simulink model "test_stimulation_visual_movie"  (Simulink 4.00)
settings: Solver=FixedStepDiscrete  SolverMode=SingleTasking  StartTime=0.0  StopTime=24  FixedStep=0.05  RelTol=1e-3
libraries: simulink3 x1, stimulation_visual_lib x1
settings Model: LastModifiedBy=bsaunder

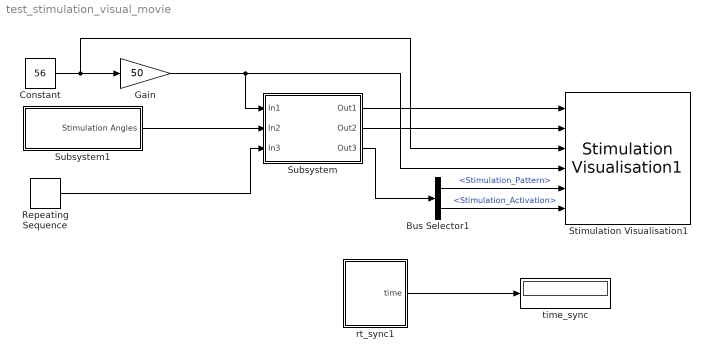
== system test_stimulation_visual_movie ==
  Bus Selector1 : BusSelector  OutputSignals=Stimulation_Pattern,Stimulation_Activation  MuxedOutput=off
  Constant : Constant  Value=56
  Gain : Gain  Gain=50  Multiplication=Element-wise(K.*u)  SaturateOnIntegerOverflow=on
  Repeating Sequence : simulink3/Sources/Repeating Sequence  rep_seq_t=[0 1 1.5 2 3]  rep_seq_y=[0.0 0.25 0.5 1.0 1.0]
  Stimulation Visualisation1 : stimulation_visual_lib/Stimulation Visualisation1  show=on  Ts=0.05
  Subsystem : Subsystem
      settings: RTWFcnNameOpts=Auto  RTWFileNameOpts=Auto
  Subsystem1 : Subsystem
      settings: RTWFcnNameOpts=Auto  RTWFileNameOpts=Auto
  rt_sync1 : Subsystem  mask{Ts=0.05}
      mask prompts: Ts "Sample Time"
      settings: RTWFcnNameOpts=Auto  RTWFileNameOpts=Auto
      mask Display: fprintf('Real\n Time\n sync')
  time_sync : Display
      settings: Format=short
  wires:
  Repeating Sequence/1 -> Subsystem/3(In3)
  Subsystem1/1(Stimulation Angles) -> Subsystem/2(In2)
  Constant/1 -> Gain/1, Stimulation Visualisation1/3
  Gain/1 -> Subsystem/1(In1), Stimulation Visualisation1/4
  Bus Selector1/1 -> Stimulation Visualisation1/5  "<Stimulation_Pattern>"
  Bus Selector1/2 -> Stimulation Visualisation1/6  "<Stimulation_Activation>"
  Subsystem/3(Out3) -> Bus Selector1/1
  Subsystem/1(Out1) -> Stimulation Visualisation1/1
  Subsystem/2(Out2) -> Stimulation Visualisation1/2
  rt_sync1/1(time) -> time_sync/1

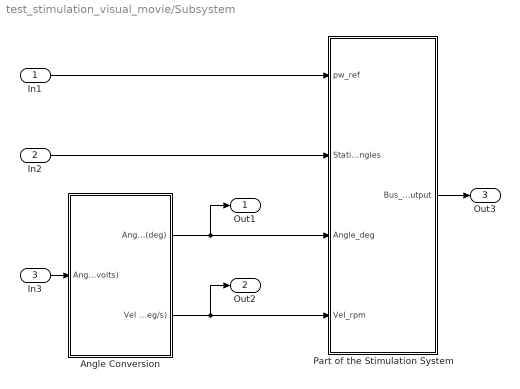
== system test_stimulation_visual_movie/Subsystem ==
  In1 : Inport  Port=1  LatchInput=off
  In2 : Inport  Port=2  LatchInput=off
  In3 : Inport  Port=3  LatchInput=off
  Angle Conversion : Subsystem
      settings: RTWFcnNameOpts=Auto  RTWFileNameOpts=Auto
  Part of the Stimulation System : Subsystem
      settings: RTWFcnNameOpts=Auto  RTWFileNameOpts=Auto
  Out1 : Outport  Port=1
  Out2 : Outport  Port=2
  Out3 : Outport  Port=3
  wires:
  Angle Conversion/1(Angle (deg)) -> Part of the Stimulation System/3(Angle_deg), Out1/1
  Angle Conversion/2(Vel (deg/s)) -> Part of the Stimulation System/4(Vel_rpm), Out2/1
  Part of the Stimulation System/1(Bus_Output) -> Out3/1
  In1/1 -> Part of the Stimulation System/1(pw_ref)
  In2/1 -> Part of the Stimulation System/2(Static Stimulation Angles)
  In3/1 -> Angle Conversion/1(Angle (0 to 1 volts))

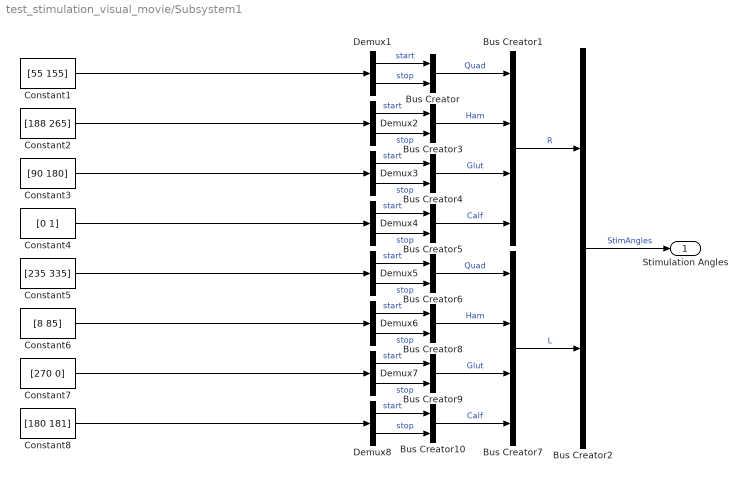
== system test_stimulation_visual_movie/Subsystem1 ==
  Bus Creator{,2..6,8..10} (9 alike) : BusCreator  Inputs=2
  Bus Creator1 : BusCreator  Inputs=4
  Bus Creator7 : BusCreator  Inputs=4
  Constant1 : Constant  Value=[55 155]
  Constant2 : Constant  Value=[188 265]
  Constant3 : Constant  Value=[90 180]
  Constant4 : Constant  Value=[0 1]
  Constant5 : Constant  Value=[235 335]
  Constant6 : Constant  Value=[8 85]
  Constant7 : Constant  Value=[270 0]
  Constant8 : Constant  Value=[180 181]
  Demux{1..8} (8 alike) : Demux  Outputs=2  BusSelectionMode=off
  Stimulation Angles : Outport  Port=1
  wires:
  Bus Creator7/1 -> Bus Creator2/2  "L"
  Constant8/1 -> Demux8/1
  Constant7/1 -> Demux7/1
  Constant6/1 -> Demux6/1
  Constant5/1 -> Demux5/1
  Bus Creator10/1 -> Bus Creator7/4  "Calf"
  Bus Creator9/1 -> Bus Creator7/3  "Glut"
  Bus Creator8/1 -> Bus Creator7/2  "Ham"
  Demux8/2 -> Bus Creator10/2  "stop"
  Demux8/1 -> Bus Creator10/1  "start"
  Demux7/2 -> Bus Creator9/2  "stop"
  Demux7/1 -> Bus Creator9/1  "start"
  Demux6/2 -> Bus Creator8/2  "stop"
  Demux6/1 -> Bus Creator8/1  "start"
  Bus Creator6/1 -> Bus Creator7/1  "Quad"
  Demux5/2 -> Bus Creator6/2  "stop"
  Demux5/1 -> Bus Creator6/1  "start"
  Constant4/1 -> Demux4/1
  Constant3/1 -> Demux3/1
  Constant2/1 -> Demux2/1
  Bus Creator5/1 -> Bus Creator1/4  "Calf"
  Bus Creator4/1 -> Bus Creator1/3  "Glut"
  Bus Creator3/1 -> Bus Creator1/2  "Ham"
  Demux4/2 -> Bus Creator5/2  "stop"
  Demux4/1 -> Bus Creator5/1  "start"
  Demux3/2 -> Bus Creator4/2  "stop"
  Demux3/1 -> Bus Creator4/1  "start"
  Demux2/2 -> Bus Creator3/2  "stop"
  Demux2/1 -> Bus Creator3/1  "start"
  Bus Creator1/1 -> Bus Creator2/1  "R"
  Bus Creator/1 -> Bus Creator1/1  "Quad"
  Demux1/2 -> Bus Creator/2  "stop"
  Demux1/1 -> Bus Creator/1  "start"
  Constant1/1 -> Demux1/1
  Bus Creator2/1 -> Stimulation Angles/1  "StimAngles"

== system test_stimulation_visual_movie/rt_sync1 ==
  S-Function : S-Function  FunctionName=sf_rtsync  Parameters=Ts  PortCounts=[]  SFunctionModules=''
  time : Outport  Port=1
  wires:
  S-Function/1 -> time/1

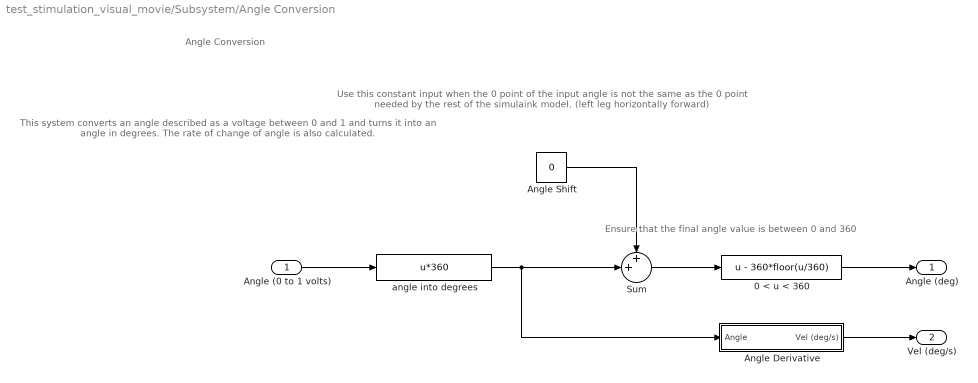
== system test_stimulation_visual_movie/Subsystem/Angle Conversion ==
  note: Angle Conversion
  note: Use this constant input
      | when the 0 point of the
      | input angle is not the same
      | as the 0 point needed by
      | the rest of the simulaink
      | model.
      | (left leg horizontally forward)
  note: Ensure that the final angle
      | value is between 0 and 360
  note: This system converts an
      | angle described as a voltage
      | between 0 and 1 and turns it
      | into an angle in degrees.
      | The rate of change of angle
      | is also calculated.
  Angle (0 to 1 volts) : Inport  Port=1  LatchInput=off
  0 < u < 360 : Fcn  Expr=u - 360*floor(u/360)
  Angle Derivative : Subsystem  mask(AngleDer){Tdf=0.5, Ts=0.05}
      mask prompts: Tdf "Filter constant"; Ts "Sampling Time"
      mask help:
      | This block calculates the angular velocity from the angle measuremet.  If the input angle is in degrees then the output velocity is in deg/s.  The block takes account of the transition from 359 deg to 0 deg or vice versa and computes the derivative based on the sample time given  The output is passed through a low pass filter based on the fliter constant also given.
      |
      | Implemented by Nils-Otto Negaard
      | Documented by Ben Saunders (17/06/2003)
      settings: RTWFcnNameOpts=Auto  RTWFileNameOpts=Auto
  Angle Shift : Constant  Value=0
  Sum : Sum  Inputs=++|  SaturateOnIntegerOverflow=on
  angle into degrees : Fcn  Expr=u*360
  Angle (deg) : Outport  Port=1
  Vel (deg/s) : Outport  Port=2
  wires:
  Angle Shift/1 -> Sum/1
  Angle Derivative/1(Vel (deg/s)) -> Vel (deg/s)/1
  Angle (0 to 1 volts)/1 -> angle into degrees/1
  0 < u < 360/1 -> Angle (deg)/1
  Sum/1 -> 0 < u < 360/1
  angle into degrees/1 -> Sum/2, Angle Derivative/1(Angle)

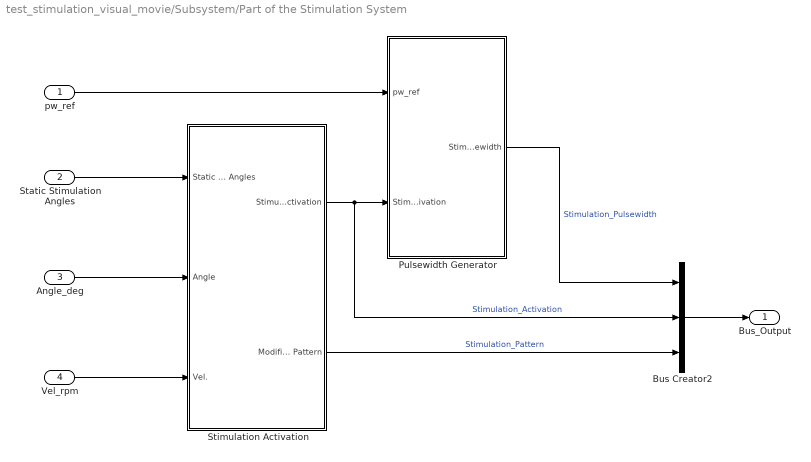
== system test_stimulation_visual_movie/Subsystem/Part of the Stimulation System ==
  pw_ref : Inport  Port=1  LatchInput=off
  Static Stimulation Angles : Inport  Port=2  LatchInput=off
  Angle_deg : Inport  Port=3  LatchInput=off
  Vel_rpm : Inport  Port=4  LatchInput=off
  Bus Creator2 : BusCreator  Inputs=3
  Pulsewidth Generator : Subsystem
      settings: RTWFcnNameOpts=Auto  RTWFileNameOpts=Auto
  Stimulation Activation : Subsystem
      settings: RTWFcnNameOpts=Auto  RTWFileNameOpts=Auto
  Bus_Output : Outport  Port=1
  wires:
  Bus Creator2/1 -> Bus_Output/1
  pw_ref/1 -> Pulsewidth Generator/1(pw_ref)
  Stimulation Activation/2(Modified Stimulation Pattern) -> Bus Creator2/3  "Stimulation_Pattern"
  Pulsewidth Generator/1(Stimulation Pulsewidth) -> Bus Creator2/1  "Stimulation_Pulsewidth"
  Vel_rpm/1 -> Stimulation Activation/3(Vel.)
  Angle_deg/1 -> Stimulation Activation/2(Angle)
  Static Stimulation Angles/1 -> Stimulation Activation/1(Static Stimulation Angles)
  Stimulation Activation/1(Stimulation Activation) -> Bus Creator2/2, Pulsewidth Generator/2(Stimulation Activation)  "Stimulation_Activation"

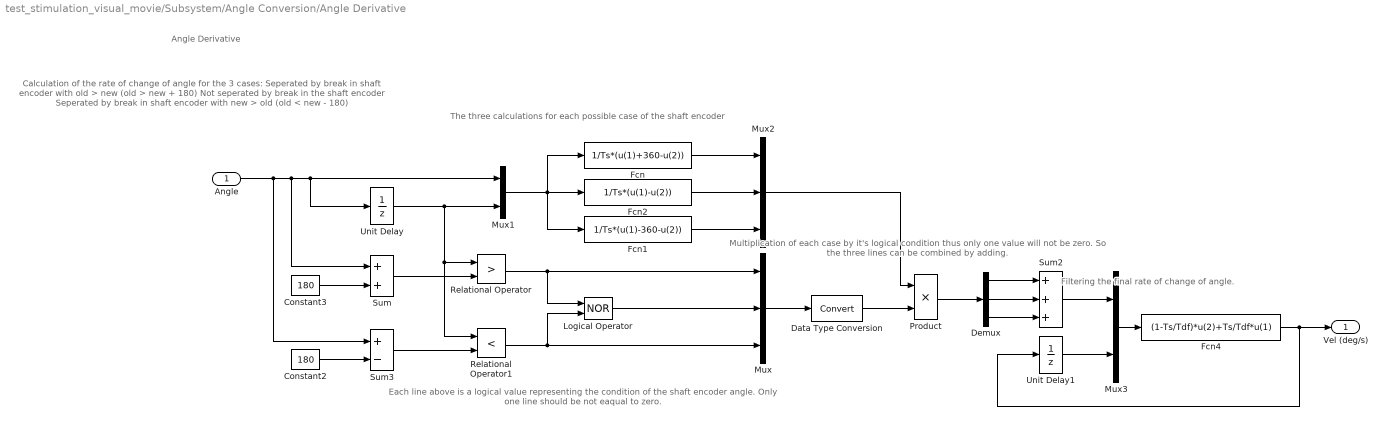
== system test_stimulation_visual_movie/Subsystem/Angle Conversion/Angle Derivative ==
  note: Angle Derivative
  note: Filtering the final rate of
      | change of angle.
  note: Multiplication of each case
      | by it's logical condition thus
      | only one value will not be zero.
      | So the three lines can be
      | combined by adding.
  note: The three calculations for each
      | possible case of the shaft encoder
  note: Each line above is a logical value
      | representing the condition of the
      | shaft encoder angle.  Only one line
      | should be not eaqual to zero.
  note: Calculation of the rate of change of angle
      | for the 3 cases:
      | Seperated by break in shaft encoder with old > new (old > new + 180)
      | Not seperated by break in the shaft encoder
      | Seperated by break in shaft encoder with new > old (old < new - 180)
  Angle : Inport  Port=1  LatchInput=off
  Constant2 : Constant  Value=180  VectorParams1D=off
  Constant3 : Constant  Value=180  VectorParams1D=off
  Data Type Conversion : DataTypeConversion  DataType=double  SaturateOnIntegerOverflow=on
  Demux : Demux  Outputs=3  BusSelectionMode=off
  Fcn : Fcn  Expr=1/Ts*(u(1)+360-u(2))
  Fcn1 : Fcn  Expr=1/Ts*(u(1)-360-u(2))
  Fcn2 : Fcn  Expr=1/Ts*(u(1)-u(2))
  Fcn4 : Fcn  Expr=(1-Ts/Tdf)*u(2)+Ts/Tdf*u(1)
  Logical Operator : Logic  Operator=NOR  Inputs=2
  Mux : Mux  Inputs=3
  Mux1 : Mux  Inputs=2
  Mux2 : Mux  Inputs=3
  Mux3 : Mux  Inputs=2
  Product : Product  Inputs=2  Multiplication=Element-wise(.*)  SaturateOnIntegerOverflow=on
  Relational Operator : RelationalOperator  Operator=>
  Relational Operator1 : RelationalOperator  Operator=<
  Sum : Sum  Inputs=++  SaturateOnIntegerOverflow=on
  Sum2 : Sum  Inputs=+++  SaturateOnIntegerOverflow=on
  Sum3 : Sum  Inputs=+-  SaturateOnIntegerOverflow=on
  Unit Delay : UnitDelay  X0=0  SampleTime=0.05
      settings: RTWStateStorageClass=Auto
  Unit Delay1 : UnitDelay  X0=0  SampleTime=Ts
      settings: RTWStateStorageClass=Auto
  Vel (deg/s) : Outport  Port=1
  wires:
  Fcn1/1 -> Mux2/3
  Fcn2/1 -> Mux2/2
  Logical Operator/1 -> Mux/2
  Sum3/1 -> Relational Operator1/2
  Constant3/1 -> Sum/2
  Angle/1 -> Unit Delay/1, Mux1/1, Sum/1, Sum3/1
  Sum2/1 -> Mux3/1
  Demux/3 -> Sum2/3
  Demux/2 -> Sum2/2
  Demux/1 -> Sum2/1
  Product/1 -> Demux/1
  Unit Delay1/1 -> Mux3/2
  Mux3/1 -> Fcn4/1
  Fcn4/1 -> Vel (deg/s)/1, Unit Delay1/1
  Mux2/1 -> Product/1
  Fcn/1 -> Mux2/1
  Mux1/1 -> Fcn2/1, Fcn1/1, Fcn/1
  Mux/1 -> Data Type Conversion/1
  Relational Operator/1 -> Mux/1, Logical Operator/1
  Relational Operator1/1 -> Mux/3, Logical Operator/2
  Constant2/1 -> Sum3/2
  Sum/1 -> Relational Operator/2
  Unit Delay/1 -> Relational Operator/1, Relational Operator1/1, Mux1/2
  Data Type Conversion/1 -> Product/2

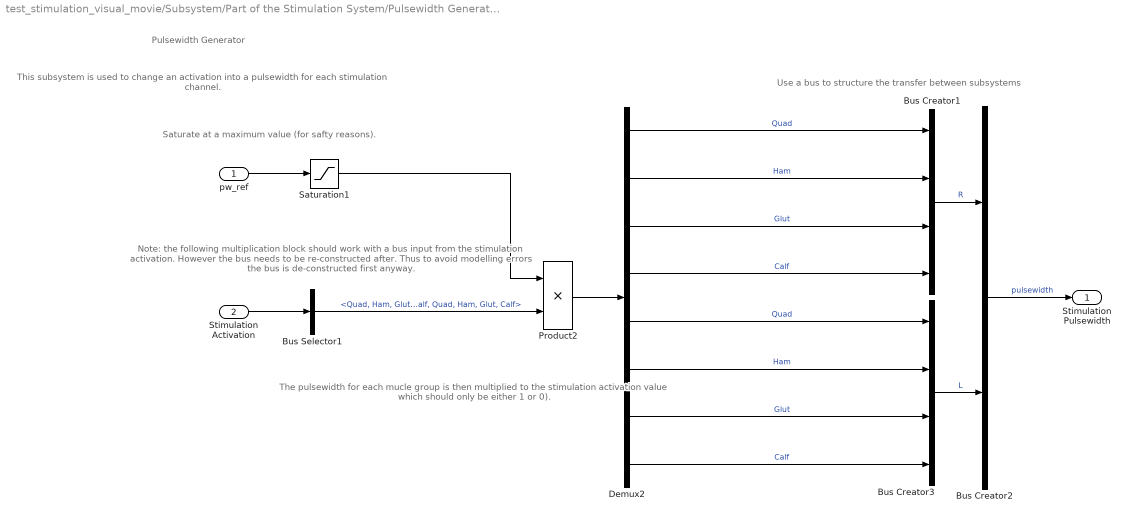
== system test_stimulation_visual_movie/Subsystem/Part of the Stimulation System/Pulsewidth Generator ==
  note: The pulsewidth for each
      | mucle group is then
      | multiplied to the stimulation
      | activation value which
      | should only be either 1 or 0).
  note: Use a bus to structure the
      | transfer between subsystems
  note: Note: the following multiplication
      | block should work with a bus input
      | from the stimulation activation.
      | However the bus needs to be
      | re-constructed after.  Thus to
      | avoid modelling errors the bus is
      | de-constructed first anyway.
  note: This subsystem is used to change
      | an activation into a pulsewidth for
      | each stimulation channel.
  note: Pulsewidth Generator
  note: Saturate at a maximum
      | value (for safty reasons).
  pw_ref : Inport  Port=1  LatchInput=off
  Stimulation Activation : Inport  Port=2  LatchInput=off
  Bus Creator1 : BusCreator  Inputs=4
  Bus Creator2 : BusCreator  Inputs=2
  Bus Creator3 : BusCreator  Inputs=4
  Bus Selector1 : BusSelector  OutputSignals=R.Quad,R.Ham,R.Glut,R.Calf,L.Quad,L.Ham,L.Glut,L.Calf  MuxedOutput=on
  Demux2 : Demux  Outputs=8  BusSelectionMode=off
  Product2 : Product  Inputs=2  Multiplication=Element-wise(.*)  SaturateOnIntegerOverflow=on
  Saturation1 : Saturate  UpperLimit=510  LowerLimit=0  LinearizeAsGain=on
  Stimulation Pulsewidth : Outport  Port=1
  wires:
  Saturation1/1 -> Product2/1
  pw_ref/1 -> Saturation1/1
  Product2/1 -> Demux2/1
  Bus Selector1/1 -> Product2/2  "<Quad, Ham, Glut, Calf, Quad, Ham, Glut, Calf>"
  Bus Creator2/1 -> Stimulation Pulsewidth/1  "pulsewidth"
  Bus Creator3/1 -> Bus Creator2/2  "L"
  Bus Creator1/1 -> Bus Creator2/1  "R"
  Demux2/1 -> Bus Creator1/1  "Quad"
  Demux2/2 -> Bus Creator1/2  "Ham"
  Demux2/3 -> Bus Creator1/3  "Glut"
  Demux2/4 -> Bus Creator1/4  "Calf"
  Demux2/5 -> Bus Creator3/1  "Quad"
  Demux2/6 -> Bus Creator3/2  "Ham"
  Demux2/7 -> Bus Creator3/3  "Glut"
  Demux2/8 -> Bus Creator3/4  "Calf"
  Stimulation Activation/1 -> Bus Selector1/1

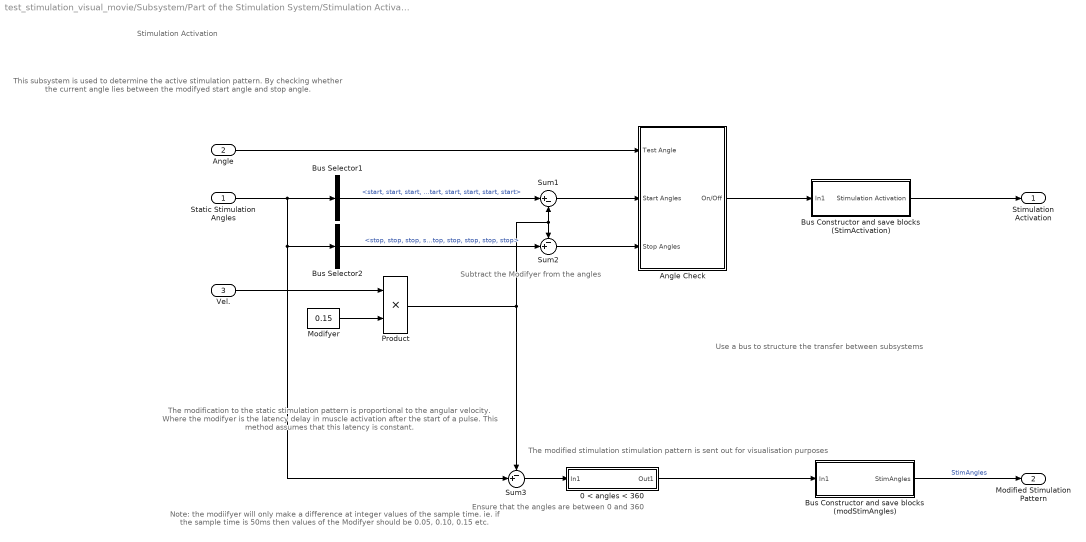
== system test_stimulation_visual_movie/Subsystem/Part of the Stimulation System/Stimulation Activation ==
  note: Use a bus to structure the
      | transfer between subsystems
  note: The modified stimulation
      | stimulation pattern is sent
      | out for visualisation purposes
  note: Note: the modiifyer will only
      | make a difference at integer
      | values of the sample time.
      | ie. if the sample time is 50ms
      | then values of the Modifyer
      | should be 0.05, 0.10, 0.15 etc.
  note: The modification to the static stimulation
      | pattern is proportional to the angular
      | velocity.  Where the modifyer is the
      | latency delay in muscle activation after
      | the start of a pulse.  This method
      | assumes that this latency is constant.
  note: Subtract the Modifyer
      | from the angles
  note: This subsystem is used to
      | determine the active stimulation
      | pattern.  By checking whether the
      | current angle lies between the modifyed
      | start angle and stop angle.
  note: Stimulation Activation
  note: Ensure that the angles are
      | between 0 and 360
  Static Stimulation Angles : Inport  Port=1  LatchInput=off
  Angle : Inport  Port=2  LatchInput=off
  Vel. : Inport  Port=3  LatchInput=off
  0 < angles < 360 : Subsystem
      settings: RTWFcnNameOpts=Auto  RTWFileNameOpts=Auto
  Angle Check : Subsystem
      settings: RTWFcnNameOpts=Auto  RTWFileNameOpts=Auto
  Bus Selector1 : BusSelector  OutputSignals=R.Quad.start,R.Ham.start,R.Glut.start,R.Calf.start,L.Quad.start,L.Ham.start,L.Glut.start,L.Calf.start  MuxedOutput=on
  Bus Selector2 : BusSelector  OutputSignals=R.Quad.stop,R.Ham.stop,R.Glut.stop,R.Calf.stop,L.Quad.stop,L.Ham.stop,L.Glut.stop,L.Calf.stop  MuxedOutput=on
  Bus Constructor and save blocks (StimActivation) : Subsystem
      settings: RTWFcnNameOpts=Auto  RTWFileNameOpts=Auto
  Bus Constructor and save blocks (modStimAngles) : Subsystem
      settings: RTWFcnNameOpts=Auto  RTWFileNameOpts=Auto
  Modifyer : Constant  Value=0.15
  Product : Product  Inputs=2  Multiplication=Element-wise(.*)  SaturateOnIntegerOverflow=on
  Sum1 : Sum  Inputs=|+-  SaturateOnIntegerOverflow=on
  Sum2 : Sum  Inputs=-+|  SaturateOnIntegerOverflow=on
  Sum3 : Sum  Inputs=-+|  SaturateOnIntegerOverflow=on
  Stimulation Activation : Outport  Port=1
  Modified Stimulation Pattern : Outport  Port=2
  wires:
  Bus Constructor and save blocks (modStimAngles)/1(StimAngles) -> Modified Stimulation Pattern/1  "StimAngles"
  Angle Check/1(On/Off) -> Bus Constructor and save blocks (StimActivation)/1(In1)
  Bus Constructor and save blocks (StimActivation)/1(Stimulation Activation) -> Stimulation Activation/1
  Modifyer/1 -> Product/2
  Vel./1 -> Product/1
  Sum2/1 -> Angle Check/3(Stop Angles)
  Sum1/1 -> Angle Check/2(Start Angles)
  Product/1 -> Sum3/1, Sum1/2, Sum2/1
  Bus Selector2/1 -> Sum2/2  "<stop, stop, stop, stop, stop, stop, stop, stop>"
  Bus Selector1/1 -> Sum1/1  "<start, start, start, start, start, start, start, start>"
  Static Stimulation Angles/1 -> Sum3/2, Bus Selector2/1, Bus Selector1/1
  0 < angles < 360/1(Out1) -> Bus Constructor and save blocks (modStimAngles)/1(In1)
  Sum3/1 -> 0 < angles < 360/1(In1)
  Angle/1 -> Angle Check/1(Test Angle)

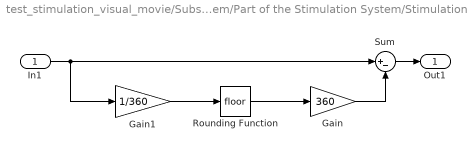
== system test_stimulation_visual_movie/Subsystem/Part of the Stimulation System/Stimulation Activation/0 < angles < 360 ==
  In1 : Inport  Port=1  LatchInput=off
  Gain : Gain  Gain=360  Multiplication=Element-wise(K.*u)  SaturateOnIntegerOverflow=on
  Gain1 : Gain  Gain=1/360  Multiplication=Element-wise(K.*u)  SaturateOnIntegerOverflow=on
  Rounding Function : Rounding  Operator=floor
  Sum : Sum  Inputs=|+-  SaturateOnIntegerOverflow=on
  Out1 : Outport  Port=1
  wires:
  In1/1 -> Sum/1, Gain1/1
  Gain1/1 -> Rounding Function/1
  Rounding Function/1 -> Gain/1
  Gain/1 -> Sum/2
  Sum/1 -> Out1/1

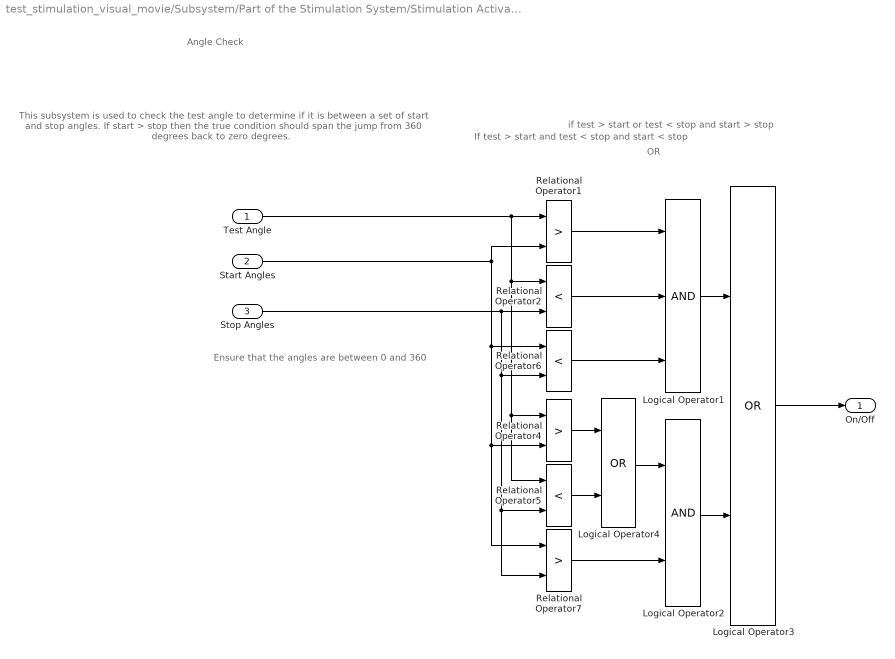
== system test_stimulation_visual_movie/Subsystem/Part of the Stimulation System/Stimulation Activation/Angle Check ==
  note: If
      |   test > start
      | and
      |   test < stop
      | and
      |   start < stop
  note: Ensure that the angles are
      | between 0 and 360
  note: if
      |   test > start
      |   or
      |   test < stop
      | and
      |   start > stop
  note: OR
  note: Angle Check
  note: This subsystem is used to check
      | the test angle to determine if it is
      | between a set of  start and stop
      | angles.  If start > stop then the
      | true condition should span the
      | jump from 360 degrees back to
      | zero degrees.
  Test Angle : Inport  Port=1  LatchInput=off
  Start Angles : Inport  Port=2  LatchInput=off
  Stop Angles : Inport  Port=3  LatchInput=off
  Logical Operator1 : Logic  Operator=AND  Inputs=3
  Logical Operator2 : Logic  Operator=AND  Inputs=2
  Logical Operator3 : Logic  Operator=OR  Inputs=2
  Logical Operator4 : Logic  Operator=OR  Inputs=2
  Relational Operator1 : RelationalOperator  Operator=>
  Relational Operator2 : RelationalOperator  Operator=<
  Relational Operator4 : RelationalOperator  Operator=>
  Relational Operator5 : RelationalOperator  Operator=<
  Relational Operator6 : RelationalOperator  Operator=<
  Relational Operator7 : RelationalOperator  Operator=>
  On/Off : Outport  Port=1
  wires:
  Relational Operator2/1 -> Logical Operator1/2
  Relational Operator1/1 -> Logical Operator1/1
  Test Angle/1 -> Relational Operator1/1, Relational Operator4/1, Relational Operator5/1, Relational Operator2/1
  Start Angles/1 -> Relational Operator1/2, Relational Operator6/1, Relational Operator4/2, Relational Operator7/1
  Stop Angles/1 -> Relational Operator6/2, Relational Operator5/2, Relational Operator7/2, Relational Operator2/2
  Relational Operator6/1 -> Logical Operator1/3
  Relational Operator7/1 -> Logical Operator2/2
  Logical Operator1/1 -> Logical Operator3/1
  Logical Operator2/1 -> Logical Operator3/2
  Logical Operator3/1 -> On/Off/1
  Relational Operator4/1 -> Logical Operator4/1
  Relational Operator5/1 -> Logical Operator4/2
  Logical Operator4/1 -> Logical Operator2/1

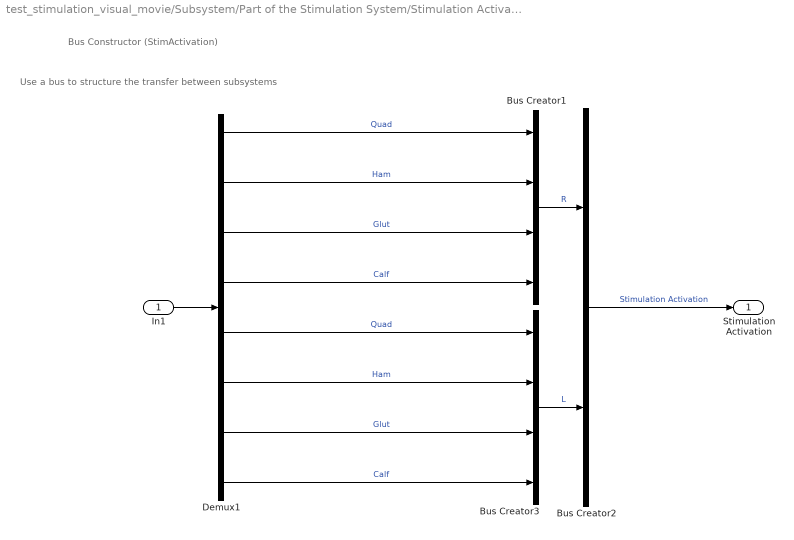
== system test_stimulation_visual_movie/Subsystem/Part of the Stimulation System/Stimulation Activation/Bus Constructor and save blocks (StimActivation) ==
  note: Bus Constructor (StimActivation)
  note: Use a bus to structure the
      | transfer between subsystems
  In1 : Inport  Port=1  LatchInput=off
  Bus Creator1 : BusCreator  Inputs=4
  Bus Creator2 : BusCreator  Inputs=2
  Bus Creator3 : BusCreator  Inputs=4
  Demux1 : Demux  Outputs=8  BusSelectionMode=off
  Stimulation Activation : Outport  Port=1
  wires:
  Bus Creator2/1 -> Stimulation Activation/1  "Stimulation Activation"
  In1/1 -> Demux1/1
  Bus Creator3/1 -> Bus Creator2/2  "L"
  Bus Creator1/1 -> Bus Creator2/1  "R"
  Demux1/1 -> Bus Creator1/1  "Quad"
  Demux1/2 -> Bus Creator1/2  "Ham"
  Demux1/3 -> Bus Creator1/3  "Glut"
  Demux1/4 -> Bus Creator1/4  "Calf"
  Demux1/5 -> Bus Creator3/1  "Quad"
  Demux1/6 -> Bus Creator3/2  "Ham"
  Demux1/7 -> Bus Creator3/3  "Glut"
  Demux1/8 -> Bus Creator3/4  "Calf"

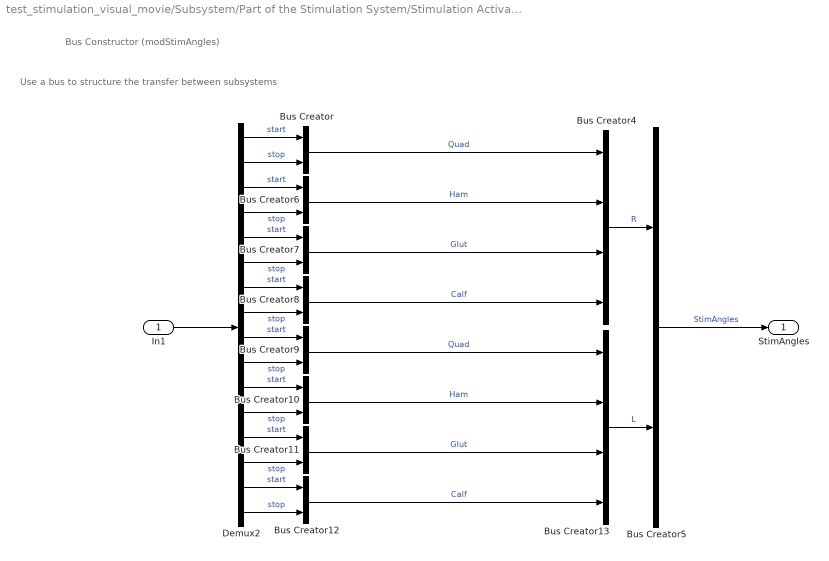
== system test_stimulation_visual_movie/Subsystem/Part of the Stimulation System/Stimulation Activation/Bus Constructor and save blocks (modStimAngles) ==
  note: Use a bus to structure the
      | transfer between subsystems
  note: Bus Constructor (modStimAngles)
  In1 : Inport  Port=1  LatchInput=off
  Bus Creator{,5..12} (9 alike) : BusCreator  Inputs=2
  Bus Creator13 : BusCreator  Inputs=4
  Bus Creator4 : BusCreator  Inputs=4
  Demux2 : Demux  Outputs=16  BusSelectionMode=off
  StimAngles : Outport  Port=1
  wires:
  Bus Creator5/1 -> StimAngles/1  "StimAngles"
  In1/1 -> Demux2/1
  Bus Creator13/1 -> Bus Creator5/2  "L"
  Bus Creator12/1 -> Bus Creator13/4  "Calf"
  Bus Creator11/1 -> Bus Creator13/3  "Glut"
  Bus Creator10/1 -> Bus Creator13/2  "Ham"
  Demux2/16 -> Bus Creator12/2  "stop"
  Demux2/15 -> Bus Creator12/1  "start"
  Demux2/14 -> Bus Creator11/2  "stop"
  Demux2/13 -> Bus Creator11/1  "start"
  Demux2/12 -> Bus Creator10/2  "stop"
  Demux2/11 -> Bus Creator10/1  "start"
  Bus Creator9/1 -> Bus Creator13/1  "Quad"
  Demux2/10 -> Bus Creator9/2  "stop"
  Demux2/9 -> Bus Creator9/1  "start"
  Bus Creator8/1 -> Bus Creator4/4  "Calf"
  Bus Creator7/1 -> Bus Creator4/3  "Glut"
  Bus Creator6/1 -> Bus Creator4/2  "Ham"
  Demux2/8 -> Bus Creator8/2  "stop"
  Demux2/7 -> Bus Creator8/1  "start"
  Demux2/6 -> Bus Creator7/2  "stop"
  Demux2/5 -> Bus Creator7/1  "start"
  Demux2/4 -> Bus Creator6/2  "stop"
  Demux2/3 -> Bus Creator6/1  "start"
  Bus Creator4/1 -> Bus Creator5/1  "R"
  Bus Creator/1 -> Bus Creator4/1  "Quad"
  Demux2/2 -> Bus Creator/2  "stop"
  Demux2/1 -> Bus Creator/1  "start"
